simulink model "check_fre"  (R2021a)
settings: Solver=VariableStepAuto  StartTime=0.0  StopTime=400000  RelTol=1e-3
undefined symbols (not defined in the file or in its folder): dtload
settings Model: Creator=PowerSystemLab  LastModifiedBy=PowerSystemLab

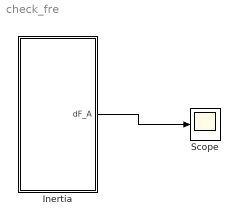
== system check_fre ==
  Inertia : Subsystem
  Scope : Scope
  wires:
  Inertia/1(dF_A) -> Scope/1

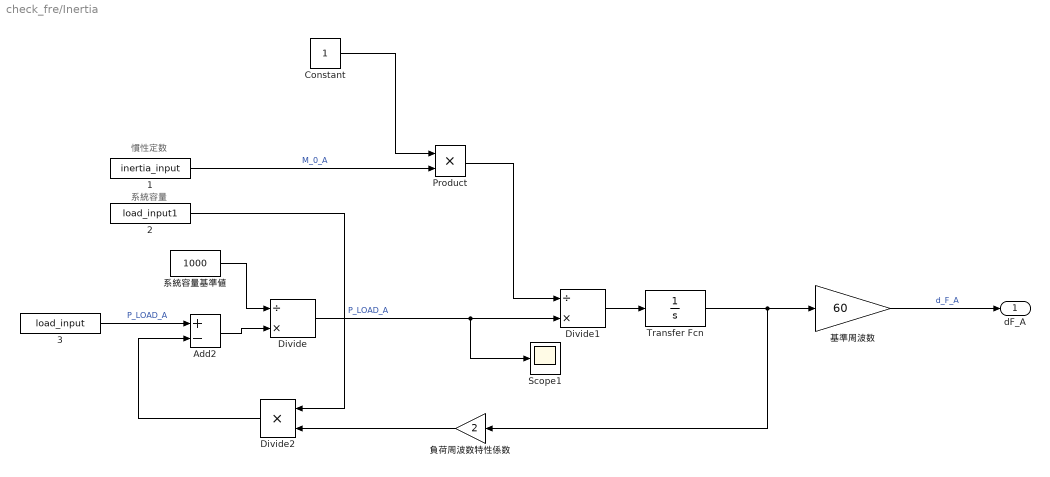
== system check_fre/Inertia ==
  note: 系統容量
  note: 慣性定数
  "  1" : FromFile  FileName=inertia_input  SampleTime=dtload
  "  2" : FromFile  FileName=load_input1  SampleTime=dtload
  "  3" : FromFile  FileName=load_input  SampleTime=dtload
  Add2 : Sum  Inputs=+-
  Constant : Constant
  Divide : Product  Inputs=/*
  Divide1 : Product  Inputs=/*
  Divide2 : Product  Inputs=**
  Product : Product
  Scope1 : Scope
  Transfer Fcn : TransferFcn  Denominator=[1 0]
  基準周波数 : Gain  Gain=60
  系統容量基準値 : Constant  Value=1000
  負荷周波数特性係数 : Gain  Gain=2
  dF_A : Outport  VectorParamsAs1DForOutWhenUnconnected=off
  wires:
  負荷周波数特性係数/1 -> Divide2/2
  Divide/1 -> Scope1/1, Divide1/2
  "  2"/1 -> Divide2/1  "P_LOAD_A"
  基準周波数/1 -> dF_A/1  "d_F_A"
  Divide1/1 -> Transfer Fcn/1
  Transfer Fcn/1 -> 負荷周波数特性係数/1, 基準周波数/1
  Add2/1 -> Divide/2
  Divide2/1 -> Add2/2
  系統容量基準値/1 -> Divide/1
  Constant/1 -> Product/1
  "  1"/1 -> Product/2  "M_0_A"
  Product/1 -> Divide1/1
  "  3"/1 -> Add2/1  "P_LOAD_A"
